simulink library "COMH"  (R2016a)
settings: Solver=ode45  StartTime=0.0  StopTime=10.0  RelTol=1e-3
undefined symbols (not defined in the file): CAL_FilterResetThd, CAL_MeasureNoise, CAL_NORTH, CAL_ProcessNoise, CAL_ROB_ERRVAL, CAL_ROBO_LENG, CAL_SAMPLE_TIME, CONST_EnableDelay, ENU_ROB_NONE
libraries: simulink x2
settings Model: Creator=oelkawok  LastModifiedBy=oelkawok
settings DataIOCC: LimitDataPoints=on
settings DebuggingCC: AllowSymbolicDim=off

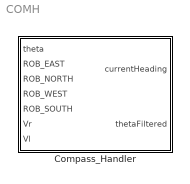
== system COMH ==
  Compass_Handler : Subsystem

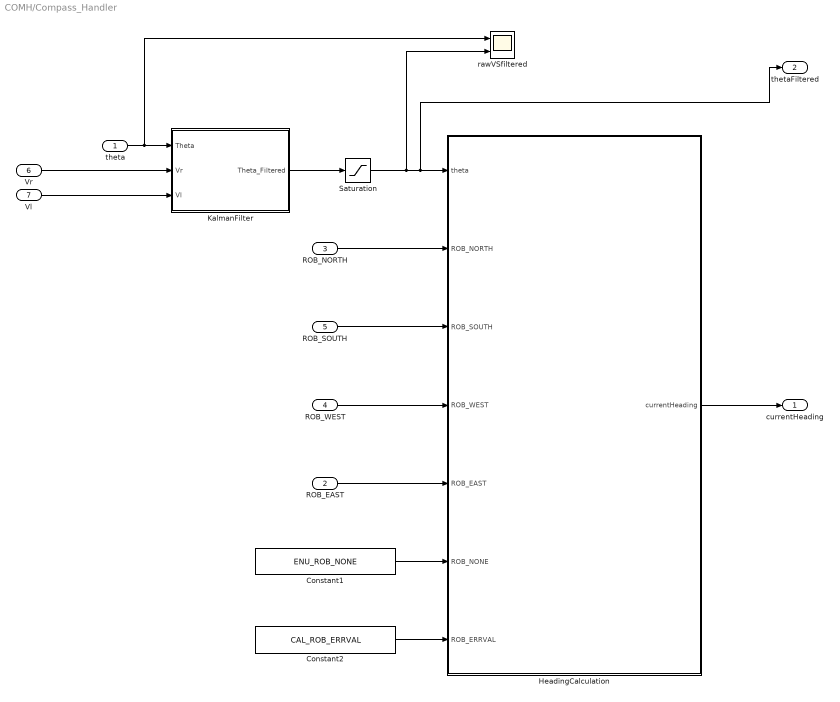
== system COMH/Compass_Handler ==
  theta : Inport
  ROB_EAST : Inport  Port=2  PortDimensions=1
  ROB_NORTH : Inport  Port=3  PortDimensions=1
  ROB_WEST : Inport  Port=4  PortDimensions=1
  ROB_SOUTH : Inport  Port=5  PortDimensions=1
  Vr : Inport  Port=6  PortDimensions=1
  Vl : Inport  Port=7  PortDimensions=1
  Constant1 : Constant  Value=ENU_ROB_NONE
  Constant2 : Constant  Value=CAL_ROB_ERRVAL
  HeadingCalculation : Stateflow chart  TreatAsAtomicUnit=on
  KalmanFilter : Subsystem
  Saturation : Saturate  UpperLimit=360  LowerLimit=0
  rawVSfiltered : Scope  NumInputPorts=2
  currentHeading : Outport
  thetaFiltered : Outport  Port=2
  wires:
  Saturation/1 -> HeadingCalculation/1(theta), thetaFiltered/1, rawVSfiltered/2
  HeadingCalculation/1(currentHeading) -> currentHeading/1
  ROB_NORTH/1 -> HeadingCalculation/2(ROB_NORTH)
  ROB_SOUTH/1 -> HeadingCalculation/3(ROB_SOUTH)
  ROB_WEST/1 -> HeadingCalculation/4(ROB_WEST)
  ROB_EAST/1 -> HeadingCalculation/5(ROB_EAST)
  Constant1/1 -> HeadingCalculation/6(ROB_NONE)
  Constant2/1 -> HeadingCalculation/7(ROB_ERRVAL)
  theta/1 -> KalmanFilter/1(Theta), rawVSfiltered/1
  Vl/1 -> KalmanFilter/3(Vl)
  Vr/1 -> KalmanFilter/2(Vr)
  KalmanFilter/1(" Theta_Filtered") -> Saturation/1

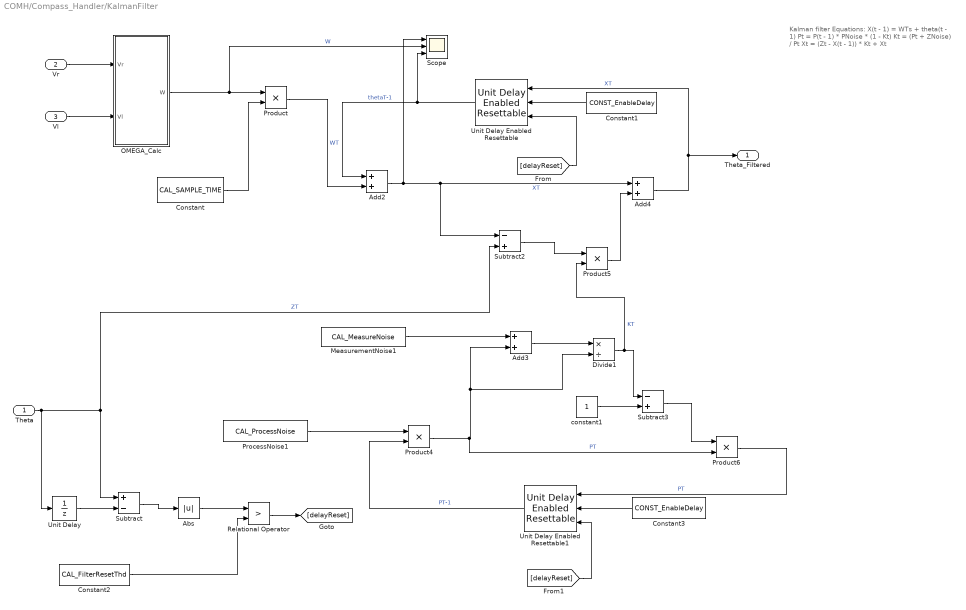
== system COMH/Compass_Handler/KalmanFilter ==
  note: Kalman filter Equations:
      | X(t - 1) = WTs + theta(t - 1)
      | Pt = P(t - 1) * PNoise * (1 - Kt)
      | Kt = (Pt + ZNoise) / Pt
      | Xt = (Zt - X(t - 1)) * Kt + Xt
  Theta : Inport
  Vr : Inport  Port=2
  Vl : Inport  Port=3
  Abs : Abs
  Add2 : Sum  OutDataTypeStr=Inherit: Same as first input
  Add3 : Sum
  Add4 : Sum  OutDataTypeStr=single
  Constant : Constant  Value=CAL_SAMPLE_TIME
  Constant1 : Constant  Value=CONST_EnableDelay
  Constant2 : Constant  Value=CAL_FilterResetThd
  Constant3 : Constant  Value=CONST_EnableDelay
  Divide1 : Product  Inputs=*/  OutDataTypeStr=Inherit: Inherit via back propagation
  MeasurementNoise1 : Constant  Value=CAL_MeasureNoise
  OMEGA_Calc : Subsystem
  ProcessNoise1 : Constant  Value=CAL_ProcessNoise
  Product : Product
  Product4 : Product  OutDataTypeStr=Inherit: Inherit via back propagation
  Product5 : Product  OutDataTypeStr=single
  Product6 : Product  OutDataTypeStr=Inherit: Inherit via back propagation
  Relational Operator : RelationalOperator  Operator=>  OutDataTypeStr=boolean
  Scope : Scope  NumInputPorts=3
  Subtract : Sum  Inputs=+-
  Subtract2 : Sum  Inputs=-+
  Subtract3 : Sum  Inputs=-+  OutDataTypeStr=Inherit: Inherit via back propagation
  Unit Delay : UnitDelay  InitialCondition=CAL_NORTH  SampleTime=-1
      settings: AttributesFormatString=%<InitialCondition>
  Unit Delay Enabled Resettable : simulink/Additional Math & Discrete/Additional Discrete/Unit Delay Enabled Resettable  vinit=360  tsamp=-1
  Unit Delay Enabled Resettable1 : simulink/Additional Math & Discrete/Additional Discrete/Unit Delay Enabled Resettable  vinit=1  tsamp=-1
  constant1 : Constant  OutDataTypeStr=single
  " Theta_Filtered" : Outport
  wires:
  Abs/1 -> Relational Operator/1
  [delayReset] -> Unit Delay Enabled Resettable1/3
  Constant3/1 -> Unit Delay Enabled Resettable1/2
  [delayReset] -> Unit Delay Enabled Resettable/3
  Relational Operator/1 -> [delayReset]
  Constant2/1 -> Relational Operator/2
  Subtract/1 -> Abs/1
  Unit Delay/1 -> Subtract/2
  Constant1/1 -> Unit Delay Enabled Resettable/2
  Add4/1 -> " Theta_Filtered"/1, Unit Delay Enabled Resettable/1  "XT"
  Product5/1 -> Add4/2
  Product6/1 -> Unit Delay Enabled Resettable1/1  "PT"
  Subtract3/1 -> Product6/1
  constant1/1 -> Subtract3/2
  Subtract2/1 -> Product5/1
  Add2/1 -> Add4/1, Subtract2/1, Scope/1  "XT"
  Divide1/1 -> Product5/2, Subtract3/1  "KT"
  Add3/1 -> Divide1/1
  MeasurementNoise1/1 -> Add3/1
  Product4/1 -> Add3/2, Divide1/2, Product6/2  "PT"
  Unit Delay Enabled Resettable1/1 -> Product4/2  "PT-1"
  ProcessNoise1/1 -> Product4/1
  Unit Delay Enabled Resettable/1 -> Add2/1, Scope/3  "thetaT-1"
  Product/1 -> Add2/2  "WT"
  Theta/1 -> Unit Delay/1, Subtract2/2, Subtract/1  "ZT"
  OMEGA_Calc/1(W) -> Product/1, Scope/2  "W"
  Constant/1 -> Product/2
  Vr/1 -> OMEGA_Calc/1(Vr)
  Vl/1 -> OMEGA_Calc/2(Vl)

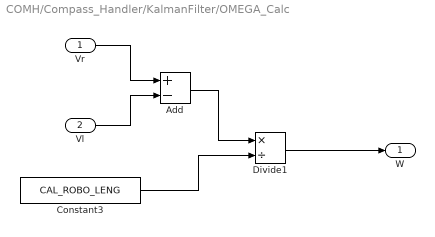
== system COMH/Compass_Handler/KalmanFilter/OMEGA_Calc ==
  Vr : Inport
  Vl : Inport  Port=2
  Add : Sum  Inputs=+-
  Constant3 : Constant  Value=CAL_ROBO_LENG
  Divide1 : Product  Inputs=*/  OutDataTypeStr=single
  W : Outport
  wires:
  Add/1 -> Divide1/1
  Divide1/1 -> W/1
  Constant3/1 -> Divide1/2
  Vr/1 -> Add/1
  Vl/1 -> Add/2

== stateflow chart COMH/Compass_Handler/HeadingCalculation ==
  state CalcHeadingEastZero
    (default) -> (junction 2)
    (junction 2) -> (junction 3) [order 1] : [(theta_OUT <= ROB_NORTH + ROB_ERRVAL) && (theta_OUT >= ROB_NORTH - ROB_ERRVAL)]//NORTH
    (junction 2) -> (junction 4) [order 2]
    (junction 3) -> (junction 17) : {currentHeading = ROB_NORTH;}
    (junction 4) -> (junction 5) [order 1] : [(theta_OUT <= ROB_SOUTH + ROB_ERRVAL) && (theta_OUT >= ROB_SOUTH - ROB_ERRVAL)]//SOUTH
    (junction 4) -> (junction 6) [order 2]
    (junction 5) -> (junction 16) : {currentHeading = ROB_SOUTH;}
    (junction 6) -> (junction 7) [order 1] : [(theta_OUT <= ROB_EAST + ROB_ERRVAL) || (theta_OUT >= 360 - ROB_ERRVAL)]//EAST
    (junction 6) -> (junction 8) [order 2]
    (junction 7) -> (junction 15) : {currentHeading = ROB_EAST;}
    (junction 8) -> (junction 9) [order 1] : [(theta_OUT <= ROB_WEST + ROB_ERRVAL) && (theta_OUT >= ROB_WEST - ROB_ERRVAL)]//WEST
    (junction 8) -> (junction 12) [order 2] : {currentHeading = ROB_NONE;}
    (junction 9) -> (junction 14) : {currentHeading = ROB_WEST;}
    (junction 14) -> (junction 12)
    (junction 15) -> (junction 14)
    (junction 16) -> (junction 15)
    (junction 17) -> (junction 16)
    (junction 12) -> (junction 18)
  state initializeDirection
    entry:
    offset = theta;
  state Calc
    entry:
    theta_OUT = theta;
    //remove for now - offset
  state CalcHeadingSouthZero
    (default) -> (junction 68)
    (junction 68) -> (junction 69) [order 1] : [(theta_OUT <= ROB_NORTH + ROB_ERRVAL) && (theta_OUT >= ROB_NORTH - ROB_ERRVAL)]//NORTH
    (junction 68) -> (junction 70) [order 2]
    (junction 69) -> (junction 80) : {currentHeading = ROB_NORTH;}
    (junction 70) -> (junction 71) [order 1] : [(theta_OUT <= ROB_SOUTH + ROB_ERRVAL) || (theta_OUT >= 360 - ROB_ERRVAL)]//SOUTH
    (junction 70) -> (junction 72) [order 2]
    (junction 71) -> (junction 79) : {currentHeading = ROB_SOUTH;}
    (junction 72) -> (junction 73) [order 1] : [(theta_OUT <= ROB_EAST + ROB_ERRVAL) && (theta_OUT >= ROB_EAST - ROB_ERRVAL)]//EAST
    (junction 72) -> (junction 74) [order 2]
    (junction 73) -> (junction 78) : {currentHeading = ROB_EAST;}
    (junction 74) -> (junction 75) [order 1] : [(theta_OUT <= ROB_WEST + ROB_ERRVAL) && (theta_OUT >= ROB_WEST - ROB_ERRVAL)]//WEST
    (junction 74) -> (junction 76) [order 2] : {currentHeading = ROB_NONE;}
    (junction 75) -> (junction 77) : {currentHeading = ROB_WEST;}
    (junction 77) -> (junction 76)
    (junction 78) -> (junction 77)
    (junction 79) -> (junction 78)
    (junction 80) -> (junction 79)
    (junction 76) -> (junction 81)
  CalcHeadingEastZero -> (junction 64) : /theta_OUT = theta;
  (junction 64) -> CalcHeadingEastZero [order 1] : [ROB_EAST == 0]
  Calc -> (junction 64) [order 3] : [hasChanged(theta)]
  CalcHeadingSouthZero -> (junction 64) : /theta_OUT = theta;
  (junction 54) -> (junction 64) : /theta_OUT = theta_OUT + 360;
  (junction 64) -> CalcHeadingSouthZero [order 2] : [ROB_SOUTH == 0]
  (junction 57) -> (junction 64) : /theta_OUT = ROB_ERRVAL;
  (junction 64) -> Calc [order 3]
  (default) -> initializeDirection
  initializeDirection -> Calc
  Calc -> (junction 54) [order 1] : [theta_OUT < 0]
  Calc -> (junction 57) [order 2] : [theta_OUT < ROB_ERRVAL]
  data: theta input; ROB_NORTH input; ROB_SOUTH input; ROB_WEST input; ROB_EAST input; ROB_NONE input; ROB_ERRVAL input; theta_OUT local int16; currentHeading output uint16; offset local int16
